simulink model "identifikacia"  (R2021a)
settings: Solver=FixedStepAuto  StartTime=0.0  StopTime=180  FixedStep=Ts  RelTol=1e-3
values from neighbouring files (symbols this model uses):
  A = [-2.68660932824  -0.00784455027611; 1  0]    [back.mat]
  a0 = -0.287462296386    [back.mat]    (also in identFit.m = pop(i,1); identFitS.m = pop(i,1); results.m = Best(1); srdce.m = 1)
  a1 = -98.4503712519    [back.mat]    (also in identFit.m = pop(i,2); identFitS.m = pop(i,2); results.m = Best(2); srdce.m = Best(1))
  a2 = -36.6448408472    [back.mat]    (also in identFit.m = pop(i,4); identFitS.m = pop(i,4); results.m = Best(4); srdce.m = Best(3))
  B = [1 0]    [back.mat]
  b0 = -94.8234712437    [back.mat]    (also in identFit.m = pop(i,3); identFitS.m = pop(i,3); results.m = Best(3); srdce.m = Best(2))
  b1 = 7.2559937066    [back.mat]    (also in identFit.m = pop(i,5); identFitS.m = pop(i,5); results.m = Best(5); srdce.m = Best(4))
  C = [-0.198008601998 2.58763495901]    [back.mat]
  D = 0    [back.mat]
  xInit = [0 48.3066591618]    [back.mat]    (also in identFit.m = [0, init/C(2)]; identFitS.m = [0, init/C(2), 0]; results.m = [0, init/C(2)])
settings Model: Creator=marko  LastModifiedBy=marko

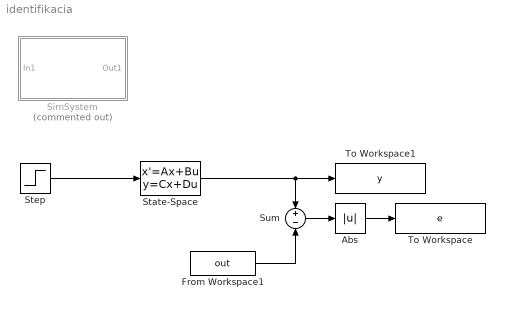
== system identifikacia ==
  Abs : Abs
  From Workspace1 : FromWorkspace  VariableName=out  Interpolate=off  OutputAfterFinalValue=Holding final value
  SimSystem : Subsystem  Commented=on
  State-Space : StateSpace  A=A  B=B  C=C  D=D  InitialCondition=xInit
  Step : Step  Time=0  Before=1  After=0  SampleTime=0
  Sum : Sum  Inputs=+|-
  To Workspace : ToWorkspace  VariableName=e  SampleTime=-1
  To Workspace1 : ToWorkspace  VariableName=y  SaveFormat=Timeseries  SampleTime=-1
  wires:
  From Workspace1/1 -> Sum/2
  Sum/1 -> Abs/1
  Abs/1 -> To Workspace/1
  Step/1 -> State-Space/1
  State-Space/1 -> To Workspace1/1, Sum/1

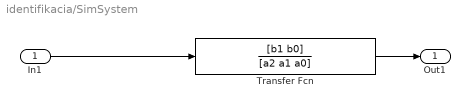
== system identifikacia/SimSystem ==
  In1 : Inport
  Transfer Fcn : TransferFcn  Numerator=[b1 b0]  Denominator=[a2 a1 a0]
  Out1 : Outport
  wires:
  In1/1 -> Transfer Fcn/1
  Transfer Fcn/1 -> Out1/1
